simulink model "bpsk_convt"  (R2018b)
settings: Solver=VariableStepAuto  StartTime=0.0  StopTime=10.0  RelTol=1e-3
libraries: commrandsrc3 x1
settings Model: Creator=DSP_27  LastModifiedBy=DSP_27

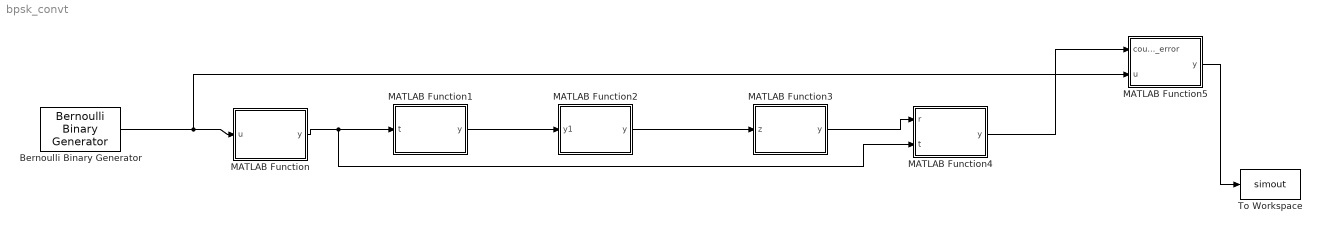
== system bpsk_convt ==
  Bernoulli Binary Generator : commrandsrc3/Bernoulli Binary Generator  ProbabilityOfZero=0.5  SeedSource=Auto  Seed=0  SampleTime=1  SamplesPerFrame=10000  OutputDataType=double  SimulateUsing=Interpreted execution
  MATLAB Function : MATLAB Function  TreatAsAtomicUnit=on
  MATLAB Function1 : MATLAB Function  TreatAsAtomicUnit=on
  MATLAB Function2 : MATLAB Function  TreatAsAtomicUnit=on
  MATLAB Function3 : MATLAB Function  TreatAsAtomicUnit=on
  MATLAB Function4 : MATLAB Function  TreatAsAtomicUnit=on
  MATLAB Function5 : MATLAB Function  TreatAsAtomicUnit=on
  To Workspace : ToWorkspace  VariableName=simout  SampleTime=-1
      settings: Save2DSignal=2-D array (concatenate along first dimension)
  wires:
  Bernoulli Binary Generator/1 -> MATLAB Function5/2(u), MATLAB Function/1(u)
  MATLAB Function/1(y) -> MATLAB Function4/2(t), MATLAB Function1/1(t)
  MATLAB Function1/1(y) -> MATLAB Function2/1(y1)
  MATLAB Function2/1(y) -> MATLAB Function3/1(z)
  MATLAB Function3/1(y) -> MATLAB Function4/1(r)
  MATLAB Function4/1(y) -> MATLAB Function5/1(count_error)
  MATLAB Function5/1(y) -> To Workspace/1

== matlab function bpsk_convt/MATLAB Function1 ==
  data: t input; y output
function y = fcn(t)

N =0;
N = length(t);
snr_db = 0;
snr_linear = zeros(length(snr_db),1);
sigma = zeros(length(snr_db),1);
 y1 = zeros(N,1);

h =zeros(N,1);
n =zeros(N,1);


h = (randn(N,1) + 1i*randn(N,1))*sqrt(1/2);  %h complex random ; ray light faded channel
n = randn(N,1);                    % noise genrated



    
snr_linear = 10.^(snr_db/10);           % converted snr to linear
sigma = 1./(snr_linear).^(1/2);                % find sigma

y1 = h.*t + sigma.*n;                 % find y = channel*bpsk_signal + sigma*noise


y = y1;

== matlab function bpsk_convt/MATLAB Function ==
  data: u input; y output
function y = fcn(u)

N=0;
N = length(u);

t = zeros(N,1);
for i = 1:N 
    if(u(i)==0)
        t(i) = -1;
    else
        t(i)= u(i);
    end
end

y = t;

== matlab function bpsk_convt/MATLAB Function2 ==
  data: y1 input; y output
function y = fcn(y1)

N =0;
N = length(y1);

h =zeros(N,1);
z = zeros(N,1);

h = (randn(N,1) + 1i*randn(N,1))*sqrt(1/2);  %h complex random ; ray light faded channel

z = y1./h;

y = z;

== matlab function bpsk_convt/MATLAB Function3 ==
  data: z input; y output
function y = fcn(z)

N = 0;
N = length(z);
r = zeros(N,1);

for i = 1:N
    if(z(i)>0)
        r(i)=1;
    else
        r(i)=-1;
    end
end


y = r;

== matlab function bpsk_convt/MATLAB Function4 ==
  data: r input; y output; t input
function y = fcn(r,t)
 
N =0;
N = length(r);

count_error=0;
for jj=1:N
    if(t(jj)~=r(jj))
        count_error=count_error+1;
%     else
%         count_error;
    end
end

 
y = count_error;

== matlab function bpsk_convt/MATLAB Function5 ==
  data: count_error input; u input; y output
function y = fcn(count_error, u)
N = 0;
N = length(u);
ber_prac = 0;


ber_prac  = count_error./N;

y = ber_prac;
